simulink model "VerificaSistemaIniziale"  (R2020b)
settings: Solver=VariableStepAuto  StartTime=0.0  StopTime=1  RelTol=1e-3
values from neighbouring files (symbols this model uses):
  theta1ldm = theta1 + Ldm_theta1.moto.data{1,1}.v    [PKM_main.m]
  theta1ldm_p = theta1_p + Ldm_theta1.moto.data{2,1}.v    [PKM_main.m]
  theta2ldm = theta2 + Ldm_theta2.moto.data{1,1}.v    [PKM_main.m]
  theta2ldm_p = theta2_p + Ldm_theta2.moto.data{2,1}.v    [PKM_main.m]
undefined symbols (not defined in the file or in its folder): C1_PLV, C2_PLV
settings Model: Creator=daniele_ravasio  LastModifiedBy=daniele_ravasio

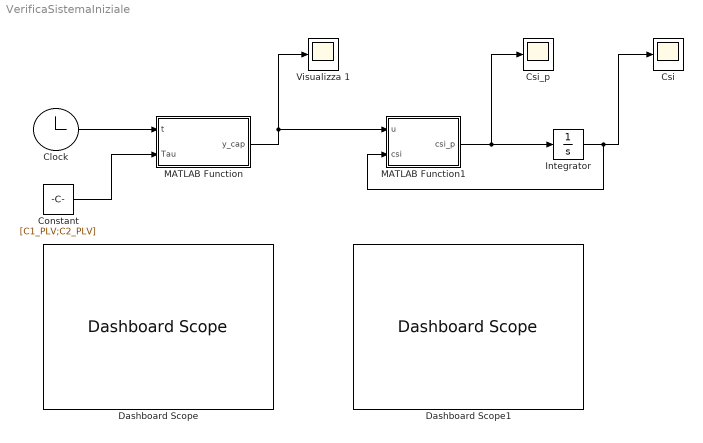
== system VerificaSistemaIniziale ==
  Clock : Clock
  Constant : Constant  Value=[C1_PLV;C2_PLV]  VectorParams1D=off
  Csi : Scope
  Csi_p : Scope
  Dashboard Scope : DashboardScope
  Dashboard Scope1 : DashboardScope
  Integrator : Integrator  InitialCondition=[theta1ldm(1,1),theta2ldm(1,1),theta1ldm_p(1,1),theta2ldm_p(1,1)]'
  MATLAB Function : MATLAB Function  TreatAsAtomicUnit=on
  MATLAB Function1 : MATLAB Function  TreatAsAtomicUnit=on
  Visualizza 1 : Scope
  wires:
  Clock/1 -> MATLAB Function/1(t)
  Constant/1 -> MATLAB Function/2(Tau)
  MATLAB Function/1(y_cap) -> MATLAB Function1/1(u), Visualizza 1/1
  Integrator/1 -> MATLAB Function1/2(csi), Csi/1
  MATLAB Function1/1(csi_p) -> Integrator/1, Csi_p/1

== matlab function VerificaSistemaIniziale/MATLAB Function ==
  data: t input; y_cap output; Tau input
function y_cap = fcn(t,Tau)


% tempo T, f(T), tempo di interpolazione (t) 
T = linspace(0,1,1000);
y_cap = [interp1(T,Tau(1,:),t);interp1(T,Tau(2,:),t)];
%y_cap(2,:) = interp1(T,Tau(2,:),t);

== matlab function VerificaSistemaIniziale/MATLAB Function1 ==
  data: u input; csi_p output; csi input
function csi_p = f(u,csi)

csi_p = F(u,csi);
